simulink library "powerlib_modelsV2"  (Simulink 6.0)
settings: Solver=ode45  SolverMode=SingleTasking  StartTime=0.0  StopTime=10.0  RelTol=1e-3
values from neighbouring files (symbols this model uses):
  Ts = get(handles.edit1,'string')    [powergui.m]
undefined symbols (not defined in the file or in its folder): A, Ac, B, Bc, C, Cc, Cs, Current, damp, Dc, Dd, DiscIntNeverNeededParam, dref, dwo, exc, F, fb, gate, GH, GHd, GI, GId, GL, GLd, H, HT, hyd, ib, ib2, io, isfinite, j, K, Kd, Kg, L, Lad, Laq, lim, LIM, Ll, Llfd, Llkd, Llkq1, Llkq2, Llr, Lls, LowerFlux, N, N2, Nb, Nb2, nb_arm, p, Par_HarmoA_pu, Par_HarmoB_pu, Par_Timing_Harmo, Par_Timing_Variation, Par_Vps, Pb ... (+57)
libraries: powerlib_extras x14
(part 8 of 11)

== system powerlib_modelsV2/Discrete/MBPSS/Transfer function for detailed model (IF) ==
  On : Inport  Port=1  LatchInput=off
  "IFpos " : Inport  Port=2  LatchInput=off
  "IFneg " : Inport  Port=3  LatchInput=off
  Switch1 : Switch  Threshold=0.5  InputSameDT=on
  Switch2 : Switch  Threshold=0.5  InputSameDT=on
  Transfer functions for detailed stabilizer : Subsystem  TreatAsAtomicUnit=on
  Transfer functions for detailed stabilizer1 : Subsystem  TreatAsAtomicUnit=on
  IFpos : Outport
  IFneg : Outport  Port=2
  wires:
  Transfer functions for detailed stabilizer/1(Out1) -> Switch1/1
  "IFpos "/1 -> Transfer functions for detailed stabilizer/1(In1), Switch1/3
  Switch1/1 -> IFpos/1
  "IFneg "/1 -> Switch2/3, Transfer functions for detailed stabilizer1/1(In1)
  Switch2/1 -> IFneg/1
  Transfer functions for detailed stabilizer1/1(Out1) -> Switch2/1
  On/1 -> Transfer functions for detailed stabilizer/Enable, Switch1/2, Switch2/2, Transfer functions for detailed stabilizer1/Enable

== system powerlib_modelsV2/Discrete/MBPSS/Transfer function for detailed model (LF) ==
  On : Inport  Port=1  LatchInput=off
  "LFpos " : Inport  Port=2  LatchInput=off
  "LFneg " : Inport  Port=3  LatchInput=off
  Switch1 : Switch  Threshold=0.5  InputSameDT=on
  Switch2 : Switch  Threshold=0.5  InputSameDT=on
  Transfer functions for detailed stabilizer : Subsystem  TreatAsAtomicUnit=on
  Transfer functions for detailed stabilizer1 : Subsystem  TreatAsAtomicUnit=on
  LFpos : Outport
  LFneg : Outport  Port=2
  wires:
  On/1 -> Transfer functions for detailed stabilizer1/Enable, Switch2/2, Switch1/2, Transfer functions for detailed stabilizer/Enable
  Transfer functions for detailed stabilizer1/1(Out1) -> Switch2/1
  Switch2/1 -> LFneg/1
  "LFneg "/1 -> Transfer functions for detailed stabilizer1/1(In1), Switch2/3
  Switch1/1 -> LFpos/1
  "LFpos "/1 -> Switch1/3, Transfer functions for detailed stabilizer/1(In1)
  Transfer functions for detailed stabilizer/1(Out1) -> Switch1/1

== system powerlib_modelsV2/Discrete/PM_synchronous_machine/abc2qd ==
  note: This subsystem converts Vab and Vbc to Vd,Vq. The sine and cosine com-
      | puted here are sent to the inverse transformation subsystem dq2abc.
  Vab,Vbc : Inport  Port=1  LatchInput=off
  the : Inport  Port=2  LatchInput=off
  Elementary Math : ElementaryMath
  Elementary Math1 : ElementaryMath  Operator=cos
  Fcn2 : Fcn  Expr=(u[4]*(2*u[1]+u[2]) + (sqrt3*u[2]*u[3])) * one_third
  Fcn3 : Fcn  Expr=(u[3]*(2*u[1]+u[2]) + (-sqrt3*u[2]*u[4])) * one_third
  Mux1 : Mux  Inputs=[ 2 2 ]
  Mux2 : Mux  Inputs=2
  Mux3 : Mux  Inputs=2
  s,c : Outport  InitialOutput=0
  vq,vd : Outport  Port=2  InitialOutput=0
  wires:
  Mux1/1 -> Fcn2/1, Fcn3/1
  Mux3/1 -> s,c/1, Mux1/2
  Fcn2/1 -> Mux2/1
  Fcn3/1 -> Mux2/2
  Mux2/1 -> vq,vd/1
  Vab,Vbc/1 -> Mux1/1
  Elementary Math/1 -> Mux3/1
  Elementary Math1/1 -> Mux3/2
  the/1 -> Elementary Math/1, Elementary Math1/1

== system powerlib_modelsV2/Discrete/PM_synchronous_machine/iq,id ==
  vq,vd : Inport  Port=1  LatchInput=off
  we : Inport  Port=2  LatchInput=off
  Demux : Demux  Outputs=2
  Mux : Mux  Inputs=2
  id : Subsystem
  iq : Subsystem
  iq,id : Outport  InitialOutput=0
  wires:
  we/1 -> iq/2(we), id/2(we)
  id/1(id) -> Mux/2, iq/3(id)
  iq/1(iq) -> Mux/1, id/1(iq)
  Demux/2 -> id/3(vd)
  Demux/1 -> iq/1(vq)
  vq,vd/1 -> Demux/1
  Mux/1 -> iq,id/1

== system powerlib_modelsV2/Discrete/PM_synchronous_machine/mec ==
  Tm : Inport  Port=1  LatchInput=off
  iq,id : Inport  Port=2  LatchInput=off
  Discrete-Time Integrator : DiscreteIntegrator  SampleTime=Ts  SaturateOnIntegerOverflow=on  ICPrevOutput=DiscIntNeverNeededParam  ICPrevScaledInput=DiscIntNeverNeededParam
  Discrete-Time Integrator1 : DiscreteIntegrator  SampleTime=Ts  SaturateOnIntegerOverflow=on  ICPrevOutput=DiscIntNeverNeededParam  ICPrevScaledInput=DiscIntNeverNeededParam
  Gain : Gain  Gain=p  SaturateOnIntegerOverflow=on
  Gain1 : Gain  Gain=1/p  SaturateOnIntegerOverflow=on
  Gain2 : Gain  Gain=1/J  SaturateOnIntegerOverflow=on
  Gain3 : Gain  Gain=F  SaturateOnIntegerOverflow=on
  Mux1 : Mux  Inputs=3
  Sum : Sum  Inputs=-+-  SaturateOnIntegerOverflow=on  InputSameDT=on
  Te : Fcn  Expr=1.5*p*(lam*u(1)+(Ld-Lq)*u(1)*u(2))
  we : Outport  InitialOutput=0
  the : Outport  Port=2  InitialOutput=0
  w,th,Te : Outport  Port=3  InitialOutput=0
  wires:
  Discrete-Time Integrator1/1 -> Gain1/1, the/1
  Gain1/1 -> Mux1/2
  iq,id/1 -> Te/1
  Gain/1 -> we/1, Discrete-Time Integrator1/1
  Discrete-Time Integrator/1 -> Mux1/1, Gain3/1, Gain/1
  Gain2/1 -> Discrete-Time Integrator/1
  Sum/1 -> Gain2/1
  Tm/1 -> Sum/1
  Te/1 -> Mux1/3, Sum/2
  Mux1/1 -> w,th,Te/1
  Gain3/1 -> Sum/3

== system powerlib_modelsV2/Discrete/PM_synchronous_machine/qd2abc ==
  s,c : Inport  Port=1  LatchInput=off
  iq,id : Inport  Port=2  LatchInput=off
  Fcn : Fcn  Expr=u[3]*u[2] + u[4]*u[1]
  Fcn1 : Fcn  Expr=(u[2]*(-u[3]-sqrt3*u[4]) + u[1]*(sqrt3*u[3]-u[4]))*0.5
  Mux : Mux  Inputs=[2,2]
  Mux2 : Mux  Inputs=3
  Sum : Sum  Orientation=down  Inputs=--  SaturateOnIntegerOverflow=on  InputSameDT=on
  is : Outport  InitialOutput=0
  wires:
  Mux/1 -> Fcn/1, Fcn1/1
  s,c/1 -> Mux/1
  iq,id/1 -> Mux/2
  Sum/1 -> Mux2/3
  Fcn/1 -> Mux2/1, Sum/2
  Fcn1/1 -> Mux2/2, Sum/1
  Mux2/1 -> is/1

== system powerlib_modelsV2/Discrete/PSS/Lead-Lag #1 ==
  In1 : Inport  Port=1  LatchInput=off
  Discrete State-Space : DiscreteStateSpace  A=Ad  B=Bd  C=Cd  D=Dd  X0=x0d  SampleTime=Ts
  Out1 : Outport
  wires:
  Discrete State-Space/1 -> Out1/1
  In1/1 -> Discrete State-Space/1

== system powerlib_modelsV2/Discrete/PSS/Lead-Lag #2 ==
  In1 : Inport  Port=1  LatchInput=off
  Discrete State-Space : DiscreteStateSpace  A=Ad  B=Bd  C=Cd  D=Dd  X0=x0d  SampleTime=Ts
  Out1 : Outport
  wires:
  Discrete State-Space/1 -> Out1/1
  In1/1 -> Discrete State-Space/1

== system powerlib_modelsV2/Discrete/PSS/Sensor  ==
  In : Inport  Port=1  LatchInput=off
  Discrete State-Space : DiscreteStateSpace  A=Ad  B=Bd  C=Cd  D=Dd  X0=x0d  SampleTime=Ts
  Out : Outport  InitialOutput=0
  wires:
  Discrete State-Space/1 -> Out/1
  In/1 -> Discrete State-Space/1

== system powerlib_modelsV2/Discrete/PSS/Wash-out  ==
  In : Inport  Port=1  LatchInput=off
  Discrete State-Space : DiscreteStateSpace  A=Ad  B=Bd  C=Cd  D=Dd  X0=x0d  SampleTime=Ts
  Out : Outport  InitialOutput=0
  wires:
  Discrete State-Space/1 -> Out/1
  In/1 -> Discrete State-Space/1

== system powerlib_modelsV2/Discrete/Three-Level Bridge/2-level GTO-IGBT Bridge  Logic (modified) ==
  note: Note 3: See Sw3 logic
  note: Diode Logic :
      | 1) Diodes are blocked when complementary GTOs are switched on
  v : Inport  Port=1  LatchInput=off
  g : Inport  Port=2  LatchInput=off
  Block12 : Inport  Port=3  LatchInput=off
  Trig12 : Inport  Port=4  LatchInput=off
  Data Type  Conversion2 : DataTypeConversion  SaturateOnIntegerOverflow=on  RndMeth=Zero
  Data Type  Conversion4 : DataTypeConversion  SaturateOnIntegerOverflow=on  RndMeth=Zero
  Demux1 : Demux  Outputs=[nb_arm nb_arm]
  Diode Logic : Subsystem
  GTO Logic : Subsystem
  G_D : Logic  Operator=OR
  G_D2 : Logic  Operator=NOT
  G_D3 : Logic  Operator=OR
  G_D4 : Logic  Operator=OR
  Gain : Gain  Orientation=up  Gain=-1  SaturateOnIntegerOverflow=on
  Gain1 : Gain  Gain=2  SaturateOnIntegerOverflow=on
  Note 3 : Logic
  Select_Block3 : Selector  Elements=Block3Elements  InputPortWidth=nb_switch
  Select_Vsw : Selector  Elements=VswElements  InputPortWidth=nb_arm*3
  Unit Delay3 : UnitDelay  SampleTime=Ts
  Unit Delay9 : UnitDelay  SampleTime=Ts
  "Vf " : Subsystem
  status : Outport
  Vf : Outport  Port=2
  Block3 : Outport  Port=3
  status_GTO : Outport  Port=4
  wires:
  G_D3/1 -> Block3/1
  Gain1/1 -> Unit Delay9/1
  G_D2/1 -> Note 3/2
  Block12/1 -> G_D2/1
  Diode Logic/1(status) -> Note 3/1
  Diode Logic/2(block) -> Select_Block3/1
  Gain/1 -> Diode Logic/1(Vak)
  v/1 -> Select_Vsw/1
  "Vf "/1(Vf) -> Gain1/1
  GTO Logic/1(status) -> G_D/2, Diode Logic/2(G), "Vf "/1(status_GTO), status_GTO/1
  g/1 -> Data Type  Conversion4/1
  Data Type  Conversion4/1 -> GTO Logic/2(G)
  Unit Delay3/1 -> status/1
  G_D/1 -> Data Type  Conversion2/1
  Data Type  Conversion2/1 -> Unit Delay3/1
  Unit Delay9/1 -> Vf/1
  G_D4/1 -> G_D/1
  Note 3/1 -> G_D4/1
  Trig12/1 -> G_D4/2
  Select_Vsw/1 -> Gain/1, GTO Logic/1(Vak)
  Select_Block3/1 -> Demux1/1
  Demux1/1 -> G_D3/1
  Demux1/2 -> G_D3/2

== system powerlib_modelsV2/Discrete/Three-Level Bridge/Input ==
  note: This block is required when the "pulses" input is not connected
  In : Inport  Port=1  LatchInput=off
  Constant : Constant
  require : Logic  OutDataTypeMode=Specify via dialog  LogicDataType=float('double')
  Out : Outport
  wires:
  Constant/1 -> require/2
  In/1 -> require/1
  require/1 -> Out/1

== system powerlib_modelsV2/Discrete/Three-Level Bridge/SubSystem ==
  note: D5, D6 : Clamping diodes
  note: - Vdc ------------
  note: N ----
  note: -[Sw3]-----
  note: |
      | |
      | |
      | [Q1 - D1]
      | |
      | |
  note: |
      | |
      | [Q2 - D2]
      | |
      | |
  note: |
      | |
      | [Q3 - D3]
      | |
      | |
  note: |
      | |
      | [Q4 - D4]
      | |
      | |
      | |
  note: -------[D5]-->-------
  note: -----<-[D6]---------
  note: ------------ A
  note: |
      | |
      | |
      | |
      | |
      | |
      | |
      | |
      | |
      | |
      | |
  note: N ----------
  note: - Vdc--------------------------
  note: + Vdc --------------------------
  note: ---------- A
  note: + Vdc ------------
  note: |
      | |
      | |
      | |
      | |
      | [Sw1]
      | |
      | |
      | |
      | |
  note: |
      | |
      | |
      | |
      | |
      | [Sw2]
      | |
      | |
      | |
      | |
  note: <======>
  note: (or B or C)
  note: (or B or C)

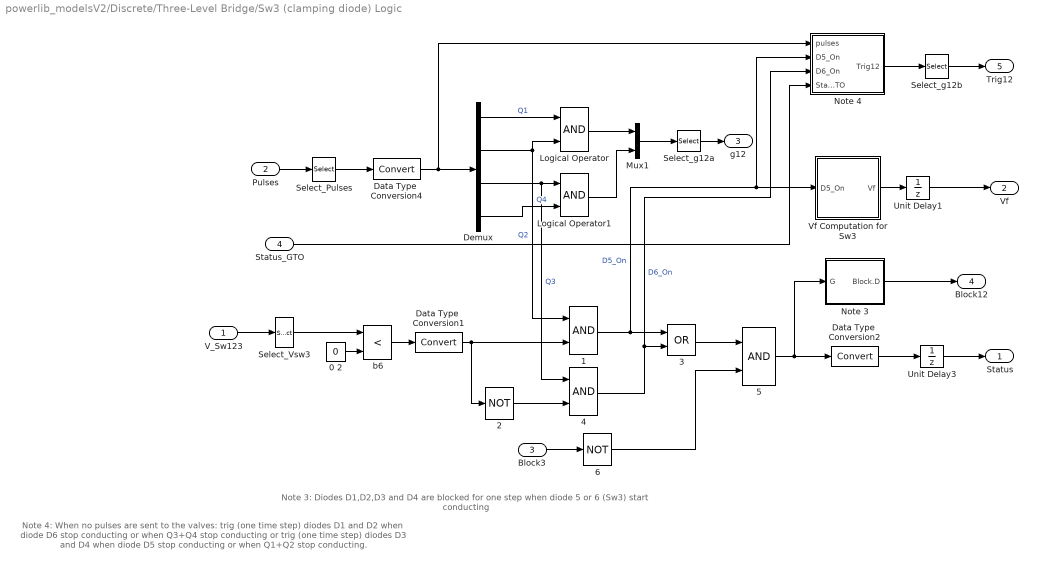
== system powerlib_modelsV2/Discrete/Three-Level Bridge/Sw3 (clamping diode) Logic ==
  note: Note 3: Diodes D1,D2,D3 and D4 are blocked for one step when diode 5 or 6 (Sw3) start conducting
  note: Note 4: When no pulses are sent to the valves:
      | trig (one time step) diodes D1 and D2 when diode D6 stop conducting or when Q3+Q4 stop conducting
      | or trig (one time step) diodes D3 and D4 when diode D5 stop conducting or when Q1+Q2 stop conducting.
  V_Sw123 : Inport  Port=1  LatchInput=off
  Pulses : Inport  Port=2  LatchInput=off
  Block3 : Inport  Port=3  LatchInput=off
  Status_GTO : Inport  Port=4  LatchInput=off
  0 2 : Constant  Value=0
  1 : Logic
  2 : Logic  Operator=NOT
  3 : Logic  Operator=OR
  4 : Logic
  5 : Logic
  6 : Logic  Operator=NOT
  Data Type  Conversion1 : DataTypeConversion  SaturateOnIntegerOverflow=on  RndMeth=Zero
  Data Type  Conversion2 : DataTypeConversion  SaturateOnIntegerOverflow=on  RndMeth=Zero
  Data Type  Conversion4 : DataTypeConversion  SaturateOnIntegerOverflow=on  RndMeth=Zero
  Demux : Demux  Outputs=[nb_arm nb_arm nb_arm nb_arm]
  Logical Operator : Logic
  Logical Operator1 : Logic
  Mux1 : Mux  Inputs=[nb_arm nb_arm]
  Note 3 : Subsystem
  Note 4 : Subsystem
  Select_Pulses : Selector  Elements=PulseElements  InputPortWidth=nb_arm*4
  Select_Vsw3 : Selector  Elements=Vsw3Elements  InputPortWidth=nb_arm*3
  Select_g12a : Selector  Elements=g12Elements  InputPortWidth=nb_arm*2
  Select_g12b : Selector  Elements=g12Elements  InputPortWidth=nb_arm*2
  Unit Delay1 : UnitDelay  SampleTime=Ts
  Unit Delay3 : UnitDelay  SampleTime=Ts
  Vf Computation for Sw3 : Subsystem
  b6 : RelationalOperator  Operator=<  InputSameDT=on
  Status : Outport
  Vf : Outport  Port=2
  g12 : Outport  Port=3
  Block12 : Outport  Port=4
  Trig12 : Outport  Port=5
  wires:
  Select_g12b/1 -> Trig12/1
  Select_g12a/1 -> g12/1
  Logical Operator/1 -> Mux1/1
  Select_Vsw3/1 -> b6/1
  5/1 -> Note 3/1(G), Data Type  Conversion2/1
  Note 3/1(Block.D) -> Block12/1
  Block3/1 -> 6/1
  Unit Delay3/1 -> Status/1
  2/1 -> 4/2
  V_Sw123/1 -> Select_Vsw3/1
  0 2/1 -> b6/2
  Pulses/1 -> Select_Pulses/1
  Mux1/1 -> Select_g12a/1
  Vf Computation for Sw3/1(Vf) -> Unit Delay1/1
  Unit Delay1/1 -> Vf/1
  Data Type  Conversion4/1 -> Demux/1, Note 4/1(pulses)
  Demux/1 -> Logical Operator/1  "Q1"
  Demux/2 -> Logical Operator/2, 1/1  "Q2"
  Demux/3 -> 4/1, Logical Operator1/1  "Q3"
  Demux/4 -> Logical Operator1/2  "Q4"
  Logical Operator1/1 -> Mux1/2
  b6/1 -> Data Type  Conversion1/1
  Data Type  Conversion1/1 -> 1/2, 2/1
  4/1 -> 3/2, Note 4/3(D6_On)  "D6_On"
  1/1 -> 3/1, Vf Computation for Sw3/1(D5_On), Note 4/2(D5_On)  "D5_On"
  3/1 -> 5/1
  6/1 -> 5/2
  Data Type  Conversion2/1 -> Unit Delay3/1
  Note 4/1(Trig12) -> Select_g12b/1
  Select_Pulses/1 -> Data Type  Conversion4/1
  Status_GTO/1 -> Note 4/4(Status_GTO)

== system powerlib_modelsV2/Discrete/asynchronous_machine/Mechanical ==
  Tm : Inport  Port=1  LatchInput=off
  phis,is : Inport  Port=2  LatchInput=off
  1\p : Gain  Gain=1/p  SaturateOnIntegerOverflow=on
  1_2H : Gain  Gain=1/(2*H)  SaturateOnIntegerOverflow=on
  1_Tb2 : Gain  Gain=1/Tb2  SaturateOnIntegerOverflow=on
  Discrete-Time Integrator : DiscreteIntegrator  InitialCondition=wmo  SampleTime=Ts  SaturateOnIntegerOverflow=on  ICPrevOutput=DiscIntNeverNeededParam  ICPrevScaledInput=DiscIntNeverNeededParam
  Discrete-Time Integrator1 : DiscreteIntegrator  InitialCondition=tho  SampleTime=Ts  SaturateOnIntegerOverflow=on  ICPrevOutput=DiscIntNeverNeededParam  ICPrevScaledInput=DiscIntNeverNeededParam
  F : Gain  Orientation=left  Gain=F  SaturateOnIntegerOverflow=on
  Mux3 : Mux  Inputs=2
  Mux4 : Mux  Inputs=3
  Product1 : Product  Inputs=1  SaturateOnIntegerOverflow=on  InputSameDT=on
  Product2 : Product  Inputs=1  SaturateOnIntegerOverflow=on  InputSameDT=on
  Selector : Selector  Elements=[1 4]  InputPortWidth=4
  Selector1 : Selector  Elements=[2 3]  InputPortWidth=4
  Sum : Sum  Inputs=-+-  SaturateOnIntegerOverflow=on  InputSameDT=on
  Sum1 : Sum  Inputs=|-+  SaturateOnIntegerOverflow=on  InputSameDT=on
  web_psb : Gain  Gain=web_psb  SaturateOnIntegerOverflow=on
  w,Te,thr : Outport
  thr,wr : Outport  Port=2
  wires:
  Discrete-Time Integrator1/1 -> Mux3/1, 1\p/1
  1\p/1 -> Mux4/3
  web_psb/1 -> Discrete-Time Integrator1/1
  Sum1/1 -> Sum/2, Mux4/2
  1_Tb2/1 -> Sum/1
  F/1 -> Sum/3
  Discrete-Time Integrator/1 -> web_psb/1, Mux4/1, Mux3/2, F/1
  1_2H/1 -> Discrete-Time Integrator/1
  Sum/1 -> 1_2H/1
  Tm/1 -> 1_Tb2/1
  Mux3/1 -> thr,wr/1
  Mux4/1 -> w,Te,thr/1
  Product1/1 -> Sum1/1
  Product2/1 -> Sum1/2
  phis,is/1 -> Selector/1, Selector1/1
  Selector1/1 -> Product2/1
  Selector/1 -> Product1/1

== system powerlib_modelsV2/Discrete/asynchronous_machine/Mutual fluxes ==
  phiqr,phidr : Inport  Port=1  LatchInput=off
  phiqs,phids : Inport  Port=2  LatchInput=off
  1\Llr : Gain  Gain=1/Llr  SaturateOnIntegerOverflow=on
  1\Llr1 : Gain  Gain=Laq  SaturateOnIntegerOverflow=on
  1\Llr2 : Gain  Gain=Lad  SaturateOnIntegerOverflow=on
  1\Lls : Gain  Gain=1/Lls  SaturateOnIntegerOverflow=on
  Demux1 : Demux  Outputs=2
  Demux2 : Demux  Outputs=2
  Mux3 : Mux  Inputs=2
  Sum : Sum  Inputs=|++  SaturateOnIntegerOverflow=on  InputSameDT=on
  Sum1 : Sum  Inputs=++|  SaturateOnIntegerOverflow=on  InputSameDT=on
  phimq,phimd : Outport
  wires:
  Mux3/1 -> phimq,phimd/1
  1\Llr2/1 -> Mux3/2
  1\Llr1/1 -> Mux3/1
  Demux1/2 -> Sum1/1
  Demux2/2 -> Sum1/2
  Demux2/1 -> Sum/2
  1\Lls/1 -> Demux2/1
  Sum/1 -> 1\Llr1/1
  Demux1/1 -> Sum/1
  1\Llr/1 -> Demux1/1
  phiqr,phidr/1 -> 1\Llr/1
  phiqs,phids/1 -> 1\Lls/1
  Sum1/1 -> 1\Llr2/1

== system powerlib_modelsV2/Discrete/asynchronous_machine/Rotor ==
  vqr,vdr : Inport  Port=1  LatchInput=off
  w-wr : Inport  Port=2  LatchInput=off
  phimq,phimd : Inport  Port=3  LatchInput=off
  1\Llr : Gain  Gain=1/Llr  SaturateOnIntegerOverflow=on
  1\Llr1 : Gain  Gain=Rr  SaturateOnIntegerOverflow=on
  1\Llr2 : Gain  Gain=1/Llr  SaturateOnIntegerOverflow=on
  1\Llr3 : Gain  Gain=Rr  SaturateOnIntegerOverflow=on
  Demux : Demux  Outputs=2
  Demux1 : Demux  Outputs=2
  Discrete-Time Integrator : DiscreteIntegrator  InitialCondition=phirqo  SampleTime=Ts  SaturateOnIntegerOverflow=on  ICPrevOutput=DiscIntNeverNeededParam  ICPrevScaledInput=DiscIntNeverNeededParam
  Discrete-Time Integrator1 : DiscreteIntegrator  InitialCondition=phirdo  SampleTime=Ts  SaturateOnIntegerOverflow=on  ICPrevOutput=DiscIntNeverNeededParam  ICPrevScaledInput=DiscIntNeverNeededParam
  Mux2 : Mux  Inputs=2
  Mux3 : Mux  Inputs=2
  Product : Product  SaturateOnIntegerOverflow=on  InputSameDT=on
  Product1 : Product  Orientation=left  SaturateOnIntegerOverflow=on  InputSameDT=on
  Sum1 : Sum  Inputs=++-||  SaturateOnIntegerOverflow=on  InputSameDT=on
  Sum2 : Sum  Inputs=+--  SaturateOnIntegerOverflow=on  InputSameDT=on
  Sum3 : Sum  Inputs=+-|  SaturateOnIntegerOverflow=on  InputSameDT=on
  Sum4 : Sum  Inputs=-+|  SaturateOnIntegerOverflow=on  InputSameDT=on
  web1 : Gain  Gain=web_psb  SaturateOnIntegerOverflow=on
  web_psb : Gain  Gain=web_psb  SaturateOnIntegerOverflow=on
  iqr,idr : Outport
  phiqr,phidr : Outport  Port=2
  wires:
  Mux3/1 -> phiqr,phidr/1
  Discrete-Time Integrator/1 -> Mux3/1, Product1/2, Sum3/1  "phiqr"
  web1/1 -> Discrete-Time Integrator1/1
  Sum1/1 -> web1/1
  w-wr/1 -> Product/2, Product1/1
  Product/1 -> Sum2/2
  web_psb/1 -> Discrete-Time Integrator/1
  Sum2/1 -> web_psb/1
  Discrete-Time Integrator1/1 -> Sum4/2, Product/1, Mux3/2
  vqr,vdr/1 -> Demux/1
  Product1/1 -> Sum1/1
  Demux/2 -> Sum1/2
  1\Llr3/1 -> Sum1/3
  1\Llr2/1 -> 1\Llr3/1, Mux2/2  "idr"
  Sum4/1 -> 1\Llr2/1
  Demux1/2 -> Sum4/1
  Mux2/1 -> iqr,idr/1
  1\Llr/1 -> Mux2/1, 1\Llr1/1  "iqr"
  1\Llr1/1 -> Sum2/3
  Sum3/1 -> 1\Llr/1
  Demux/1 -> Sum2/1
  Demux1/1 -> Sum3/2
  phimq,phimd/1 -> Demux1/1

== system powerlib_modelsV2/Discrete/asynchronous_machine/Stator ==
  phimq,phimd : Inport  Port=1  LatchInput=off
  vqs,vds : Inport  Port=2  LatchInput=off
  w : Inport  Port=3  LatchInput=off
  1\Llr : Gain  Gain=1/Lls  SaturateOnIntegerOverflow=on
  1\Llr1 : Gain  Gain=Rs  SaturateOnIntegerOverflow=on
  1\Llr2 : Gain  Gain=1/Lls  SaturateOnIntegerOverflow=on
  1\Llr3 : Gain  Gain=Rs  SaturateOnIntegerOverflow=on
  Demux : Demux  Outputs=2
  Demux1 : Demux  Outputs=2
  Discrete-Time Integrator : DiscreteIntegrator  InitialCondition=phisqo  SampleTime=Ts  SaturateOnIntegerOverflow=on  ICPrevOutput=DiscIntNeverNeededParam  ICPrevScaledInput=DiscIntNeverNeededParam
  Discrete-Time Integrator1 : DiscreteIntegrator  InitialCondition=phisdo  SampleTime=Ts  SaturateOnIntegerOverflow=on  ICPrevOutput=DiscIntNeverNeededParam  ICPrevScaledInput=DiscIntNeverNeededParam
  Mux2 : Mux  Inputs=2
  Mux3 : Mux  Inputs=2
  Mux4 : Mux  Inputs=2
  Product : Product  SaturateOnIntegerOverflow=on  InputSameDT=on
  Product1 : Product  SaturateOnIntegerOverflow=on  InputSameDT=on
  Sum1 : Sum  Inputs=++-||  SaturateOnIntegerOverflow=on  InputSameDT=on
  Sum2 : Sum  Inputs=--+  SaturateOnIntegerOverflow=on  InputSameDT=on
  Sum3 : Sum  Inputs=-+  SaturateOnIntegerOverflow=on  InputSameDT=on
  Sum4 : Sum  Inputs=+-|  SaturateOnIntegerOverflow=on  InputSameDT=on
  web1 : Gain  Gain=web_psb  SaturateOnIntegerOverflow=on
  web_psb : Gain  Gain=web_psb  SaturateOnIntegerOverflow=on
  phiqs,phids : Outport
  iqs,ids : Outport  Port=2
  phis,is : Outport  Port=3
  wires:
  phimq,phimd/1 -> Demux1/1
  Demux1/1 -> Sum4/2
  Sum4/1 -> 1\Llr/1
  1\Llr/1 -> Mux2/1, 1\Llr1/1  "iqs"
  1\Llr1/1 -> Sum2/1
  vqs,vds/1 -> Demux/1
  Sum2/1 -> web_psb/1
  Demux/1 -> Sum2/3
  Product/1 -> Sum2/2
  web_psb/1 -> Discrete-Time Integrator/1
  Discrete-Time Integrator/1 -> Mux3/1, Product1/2, Sum4/1
  Mux2/1 -> iqs,ids/1, Mux4/2
  w/1 -> Product/1, Product1/1
  Demux1/2 -> Sum3/1
  Sum3/1 -> 1\Llr2/1
  1\Llr2/1 -> 1\Llr3/1, Mux2/2  "ids"
  1\Llr3/1 -> Sum1/3
  web1/1 -> Discrete-Time Integrator1/1
  Sum1/1 -> web1/1
  Discrete-Time Integrator1/1 -> Product/2, Sum3/2, Mux3/2
  Demux/2 -> Sum1/2
  Product1/1 -> Sum1/1
  Mux3/1 -> phiqs,phids/1, Mux4/1
  Mux4/1 -> phis,is/1

== system powerlib_modelsV2/Discrete/asynchronous_machine/abc2qd ==
  v : Inport  Port=1  LatchInput=off
  sin,cos : Inport  Port=2  LatchInput=off
  1_Vb : Gain  Gain=1/Vb  SaturateOnIntegerOverflow=on
  Constant : Constant  Orientation=down  Value=ctrl==1
  Constant1 : Constant  Orientation=down  Value=ctrl==2
  Constant2 : Constant  Orientation=down  Value=ctrl==3
  Constant3 : Constant  Orientation=down  Value=ctrl
  Constant4 : Constant  Orientation=left  Value=ctrl
  Multiport Switch : MultiPortSwitch  Inputs=3  InputSameDT=on
  Multiport Switch1 : MultiPortSwitch  Inputs=3  InputSameDT=on
  Mux : Mux  Inputs=2
  Rotor reference frame : Subsystem  TreatAsAtomicUnit=on
      mask Display: disp('Rotor\nreference\nframe')
  Stationary reference frame : Subsystem  TreatAsAtomicUnit=on
      mask Display: disp('Stationary\nreference\nframe')
  Synchronous reference frame : Subsystem  TreatAsAtomicUnit=on
      mask Display: disp('Synchronous\nreference\nframe')
  transit : Subsystem
  vqr,vdr : Outport
  vqs,vds : Outport  Port=2
  wires:
  transit/1(vr,vs) -> 1_Vb/1
  Constant4/1 -> Multiport Switch1/1
  Constant3/1 -> Multiport Switch/1
  1_Vb/1 -> Mux/1
  Mux/1 -> Synchronous reference frame/1(In1), Stationary reference frame/1(In1), Rotor reference frame/1(In1)
  sin,cos/1 -> Mux/2
  Multiport Switch/1 -> vqr,vdr/1
  Synchronous reference frame/2(vqs,vds) -> Multiport Switch1/4
  Stationary reference frame/2(vqs,vds) -> Multiport Switch1/3
  Rotor reference frame/2(vqs,vds) -> Multiport Switch1/2
  Synchronous reference frame/1(vqr,vdr) -> Multiport Switch/4
  Stationary reference frame/1(vqr,vdr) -> Multiport Switch/3
  Rotor reference frame/1(vqr,vdr) -> Multiport Switch/2
  Multiport Switch1/1 -> vqs,vds/1
  Constant2/1 -> Synchronous reference frame/Enable
  Constant1/1 -> Stationary reference frame/Enable
  Constant/1 -> Rotor reference frame/Enable
  v/1 -> transit/1(vu)

== system powerlib_modelsV2/Discrete/asynchronous_machine/dq2abc ==
  sin,cos : Inport  Port=1  LatchInput=off
  iqr,idr : Inport  Port=2  LatchInput=off
  iqs,ids : Inport  Port=3  LatchInput=off
  Constant : Constant  Orientation=down  Value=ctrl==1
  Constant1 : Constant  Orientation=down  Value=ctrl==2
  Constant2 : Constant  Orientation=down  Value=ctrl==3
  Constant3 : Constant  Orientation=down  Value=ctrl
  Constant4 : Constant  Orientation=left  Value=ctrl
  Multiport Switch : MultiPortSwitch  Inputs=3  InputSameDT=on
  Multiport Switch1 : MultiPortSwitch  Inputs=3  InputSameDT=on
  Mux : Mux  Inputs=3
  Mux1 : Mux  Inputs=2
  Mux2 : Mux  Inputs=2
  Mux3 : Mux  Inputs=2
  Rotor reference frame : Subsystem  TreatAsAtomicUnit=on
      mask Display: disp('Rotor\nreference\nframe')
  Selector : Selector  Elements=elements2  InputPortWidth=4
  Stationary reference frame : Subsystem  TreatAsAtomicUnit=on
      mask Display: disp('Stationary\nreference\nframe')
  Sum2 : Sum  Inputs=-  SaturateOnIntegerOverflow=on  InputSameDT=on
  Sum3 : Sum  Inputs=-  SaturateOnIntegerOverflow=on  InputSameDT=on
  Synchronous reference frame : Subsystem  TreatAsAtomicUnit=on
      mask Display: disp('Synchronous\nreference\nframe')
  ib : Gain  Gain=ib  SaturateOnIntegerOverflow=on
  irab,isab : Outport
  irabc : Outport  Port=2
  isabc : Outport  Port=3
  wires:
  Selector/1 -> irab,isab/1
  ib/1 -> Selector/1
  Mux3/1 -> isabc/1
  Sum3/1 -> Mux3/2
  Constant4/1 -> Multiport Switch1/1
  Constant3/1 -> Multiport Switch/1
  Mux1/1 -> ib/1
  Rotor reference frame/2(isa,isb) -> Multiport Switch1/2
  sin,cos/1 -> Mux/3
  Sum2/1 -> Mux2/2
  Multiport Switch1/1 -> Mux3/1, Sum3/1, Mux1/2
  Mux2/1 -> irabc/1
  Multiport Switch/1 -> Sum2/1, Mux1/1, Mux2/1
  iqr,idr/1 -> Mux/1
  iqs,ids/1 -> Mux/2
  Mux/1 -> Synchronous reference frame/1(In1), Stationary reference frame/1(In1), Rotor reference frame/1(In1)
  Synchronous reference frame/2(isa,isb) -> Multiport Switch1/4
  Stationary reference frame/2(isa,isb) -> Multiport Switch1/3
  Synchronous reference frame/1(ira,irb) -> Multiport Switch/4
  Stationary reference frame/1(ira,irb) -> Multiport Switch/3
  Rotor reference frame/1(ira,irb) -> Multiport Switch/2
  Constant2/1 -> Synchronous reference frame/Enable
  Constant1/1 -> Stationary reference frame/Enable
  Constant/1 -> Rotor reference frame/Enable

== system powerlib_modelsV2/Discrete/asynchronous_machine/sin,cos ==
  thr,wr : Inport  Port=1  LatchInput=off
  Constant : Constant  Orientation=down  Value=ctrl<3
  Constant1 : Constant  Value=ctrl
  Constant2 : Constant  Value=0
  Constant3 : Constant  Orientation=down  Value=ctrl==3
  Constant4 : Constant  Value=ctrl
  Constant5 : Constant  Value=0
  Constant6 : Constant
  Gain : Gain  Gain=-1  SaturateOnIntegerOverflow=on
  Multiport Switch : MultiPortSwitch  Inputs=3  InputSameDT=on
  Multiport Switch1 : MultiPortSwitch  Inputs=3  InputSameDT=on
  Selector : Selector  InputPortWidth=2
  Selector1 : Selector  Elements=2  InputPortWidth=2
  Switch : Switch  Threshold=0.5  InputSameDT=on
  sin(beta),cos(beta),sin(th),cos(th) : Subsystem  TreatAsAtomicUnit=on
  sin(thr),cos(thr) : Subsystem  TreatAsAtomicUnit=on
  sin,cos : Outport
  w-wr : Outport  Port=2
  w : Outport  Port=3
  wires:
  Constant/1 -> sin(thr),cos(thr)/Enable, Switch/2
  thr,wr/1 -> Selector/1, sin(beta),cos(beta),sin(th),cos(th)/1(thr,wr), Selector1/1
  Selector/1 -> sin(thr),cos(thr)/1(thr)
  Switch/1 -> sin,cos/1
  Constant3/1 -> sin(beta),cos(beta),sin(th),cos(th)/Enable
  sin(beta),cos(beta),sin(th),cos(th)/2(we-wr) -> Multiport Switch/4
  Constant1/1 -> Multiport Switch/1
  Constant2/1 -> Multiport Switch/2
  Multiport Switch/1 -> w-wr/1
  sin(thr),cos(thr)/1(sin(thr),cos(thr)) -> Switch/1
  sin(beta),cos(beta),sin(th),cos(th)/1("sin(beta),cos(beta), sin(th),cos(th)") -> Switch/3
  Gain/1 -> Multiport Switch/3  "-wr"
  Selector1/1 -> Gain/1, Multiport Switch1/2
  Constant4/1 -> Multiport Switch1/1
  Constant5/1 -> Multiport Switch1/3
  Constant6/1 -> Multiport Switch1/4
  Multiport Switch1/1 -> w/1

== system powerlib_modelsV2/Discrete/hysteresis_transformer/Hysteresis ( always in SI ) ==
  In1 : Inport  Port=1  LatchInput=off
  Hysteresis main loop + Saturation (Lower Part) : Lookup  DialogController=Simulink.DDGSource  InputValues=LowerFlux  OutputValues=Current  SaturateOnIntegerOverflow=on
  Hysteresis main loop + Saturation. (Upper Part) : Lookup  DialogController=Simulink.DDGSource  InputValues=UpperFlux  OutputValues=Current  SaturateOnIntegerOverflow=on
  Memory : Memory
  Memory1 : Memory  Orientation=down
  SI conversion2 : Gain  Gain=ib  SaturateOnIntegerOverflow=on
  Selector : Selector  Elements=2  InputPortWidth=2
  Selector1 : Selector  InputPortWidth=2
  Sign : Signum
  Sum : Sum  Inputs=|+-  SaturateOnIntegerOverflow=on  InputSameDT=on
  Switch1 : Switch  InputSameDT=on
  Switch2 : Switch  Threshold=1.5  InputSameDT=on
  Tr : Display
  pu conversion : Gain  Gain=fb  SaturateOnIntegerOverflow=on
  sfun_psbtransfosat : S-Function  FunctionName=sfun_test  Parameters=fluxinit*fb,HT,indice,Ts,Tolerances,initialslope
  Out1 : Outport
  wires:
  Memory1/1 -> pu conversion/1
  Hysteresis main loop + Saturation (Lower Part)/1 -> Switch1/1  "courbe principale + Saturation, partie du bas, le flux est en monte, donc sens positif"
  In1/1 -> Hysteresis main loop + Saturation (Lower Part)/1, Memory/1, Sum/1, Memory1/1, Hysteresis main loop + Saturation. (Upper Part)/1
  Hysteresis main loop + Saturation. (Upper Part)/1 -> Switch1/3  "courbe principale + Saturation, partie superieure, le flux est en descente, donc sens negatif"
  Memory/1 -> Sum/2  "precedent"
  Sign/1 -> Switch1/2  "sens du flux"
  pu conversion/1 -> sfun_psbtransfosat/1
  sfun_psbtransfosat/1 -> Selector/1, Selector1/1
  Switch2/1 -> Out1/1
  Switch1/1 -> Switch2/3
  Selector/1 -> Switch2/2, Tr/1  "Tr"
  Selector1/1 -> SI conversion2/1
  SI conversion2/1 -> Switch2/1  "Boucles internes"
  Sum/1 -> Sign/1

== system powerlib_modelsV2/Discrete/simplified_sync_mach/Subsystem ==
  i : Inport  Port=1  LatchInput=off
  v : Inport  Port=2  LatchInput=off
  e : Inport  Port=3  LatchInput=off
  theta : Inport  Port=4  LatchInput=off
  wm : Inport  Port=5  LatchInput=off
  Pe : Inport  Port=6  LatchInput=off
  Gain : Gain  Gain=[ ib2*ones(3,1); Vb3*ones(6,1); 1; Nb; Pb ]  SaturateOnIntegerOverflow=on
  Mux : Mux  Inputs=[ 3 3 3 1 1 1 ]
  * : Outport  InitialOutput=0
  wires:
  i/1 -> Mux/1
  v/1 -> Mux/2
  e/1 -> Mux/3
  theta/1 -> Mux/4
  wm/1 -> Mux/5
  Pe/1 -> Mux/6
  Mux/1 -> Gain/1
  Gain/1 -> */1

== system powerlib_modelsV2/Discrete/simplified_sync_mach/Vt ==
  note: This subsystem either converts 2 line-to-line voltages to 3 line-to-neutral voltages (internal neutral)
      | and computes floating neutral voltage or directly passes Van,Vbn,Vcn if 4-wire connection.
  V : Inport  Port=1  LatchInput=off
  1_Vb : Gain  Gain=1/Vb  SaturateOnIntegerOverflow=on
  Constant : Constant  Orientation=down  Value=v6==1
  Constant1 : Constant  Value=0
  Constant2 : Constant  Value=0
  Data Type  Conversion : DataTypeConversion  Orientation=left  SaturateOnIntegerOverflow=on  RndMeth=Zero
  Data Type  Conversion1 : DataTypeConversion  SaturateOnIntegerOverflow=on  RndMeth=Zero
  Fcn : Fcn  Expr=u[1]
  Fcn1 : Fcn  Expr=u[2]
  Fcn2 : Fcn  Expr=u[3]
  Gain : Gain  Gain=1/3  SaturateOnIntegerOverflow=on
  LL2LN : Subsystem  TreatAsAtomicUnit=on
  Logical Operator : Logic  Operator=NOT
  Mux : Mux  Inputs=2
  Mux1 : Mux  Inputs=3
  Product : Product  SaturateOnIntegerOverflow=on  InputSameDT=on
  Sum : Sum  Inputs=+  SaturateOnIntegerOverflow=on  InputSameDT=on
  Sum1 : Sum  Inputs=|++  SaturateOnIntegerOverflow=on  InputSameDT=on
  Switch2 : Switch  Threshold=0.5  InputSameDT=on
  Vn : Outport  InitialOutput=0
  Vabc : Outport  Port=2  InitialOutput=0
  wires:
  Data Type  Conversion1/1 -> Product/1
  Logical Operator/1 -> Data Type  Conversion1/1
  Data Type  Conversion/1 -> Logical Operator/1
  1_Vb/1 -> Mux/1, LL2LN/1(In1)
  V/1 -> 1_Vb/1
  Product/1 -> Sum1/2
  Mux1/1 -> Product/2
  Fcn2/1 -> Mux1/3
  Fcn1/1 -> Mux1/2
  Fcn/1 -> Mux1/1
  Mux/1 -> Fcn2/1, Fcn1/1, Fcn/1
  Constant1/1 -> Mux/2
  Sum1/1 -> Vabc/1
  LL2LN/1(Out1) -> Sum1/1, Sum/1
  Constant/1 -> Data Type  Conversion/1, LL2LN/Enable, Switch2/2
  Switch2/1 -> Vn/1
  Constant2/1 -> Switch2/3
  Gain/1 -> Switch2/1
  Sum/1 -> Gain/1

== system powerlib_modelsV2/Discrete/simplified_sync_mach/Z ==
  note: This subsystem models the internal impedance of
      | the machine, which consists of  a series RL circuit.
  e : Inport  Port=1  LatchInput=off
  v : Inport  Port=2  LatchInput=off
  1/L : Gain  Gain=web_psb/L  SaturateOnIntegerOverflow=on
  Discrete-Time Integrator : DiscreteIntegrator  IntegratorMethod=Integration: Trapezoidal  InitialCondition=io  SampleTime=Ts  SaturateOnIntegerOverflow=on  ICPrevOutput=DiscIntNeverNeededParam  ICPrevScaledInput=DiscIntNeverNeededParam
  R : Gain  Orientation=left  Gain=R  SaturateOnIntegerOverflow=on
  Sum5 : Sum  Inputs=-+-  SaturateOnIntegerOverflow=on  InputSameDT=on
  Unit Delay : UnitDelay  X0=io  SampleTime=Ts
  i : Outport  InitialOutput=0
  wires:
  e/1 -> Sum5/2
  R/1 -> Sum5/1
  Sum5/1 -> 1/L/1
  v/1 -> Sum5/3
  1/L/1 -> Discrete-Time Integrator/1
  Discrete-Time Integrator/1 -> Unit Delay/1
  Unit Delay/1 -> R/1, i/1

== system powerlib_modelsV2/Discrete/simplified_sync_mach/gen ==
  note: This subsystem generates the 3 line-to-neutral voltages inside the machine.
  theta : Inport  Port=1  LatchInput=off
  E : Inport  Port=2  LatchInput=off
  Vn : Inport  Port=3  LatchInput=off
  1_Vb2 : Gain  Gain=1/Vb2  SaturateOnIntegerOverflow=on
  Mux : Mux  Inputs=3
  Product : Product  SaturateOnIntegerOverflow=on  InputSameDT=on
  Sum : Sum  Inputs=|++  SaturateOnIntegerOverflow=on  InputSameDT=on
  Sum1 : Sum  Orientation=down  Inputs=--  SaturateOnIntegerOverflow=on  InputSameDT=on
  rem(wt,2pi) : Fcn  Expr=rem(u[1],2*pi)
  sin(a) : Fcn  Expr=sin(u)
  sin(b) : Fcn  Expr=sin(u-pi23)
  e : Outport  InitialOutput=0
  wires:
  Sum/1 -> e/1
  Product/1 -> Sum/1
  Mux/1 -> Product/1
  Vn/1 -> Sum/2
  1_Vb2/1 -> Product/2
  E/1 -> 1_Vb2/1
  sin(b)/1 -> Mux/2, Sum1/1
  Sum1/1 -> Mux/3
  sin(a)/1 -> Mux/1, Sum1/2
  theta/1 -> rem(wt,2pi)/1
  rem(wt,2pi)/1 -> sin(b)/1, sin(a)/1

== system powerlib_modelsV2/Discrete/simplified_sync_mach/mechanics ==
  Pm : Inport  Port=1  LatchInput=off
  Pe : Inport  Port=2  LatchInput=off
  1_(2*H) : Gain  Gain=1/(2*H)  SaturateOnIntegerOverflow=on
  1_Pb : Gain  Gain=1/Pb  SaturateOnIntegerOverflow=on
  Discrete-Time Integrator : DiscreteIntegrator  IntegratorMethod=Integration: Trapezoidal  InitialCondition=dwo  SampleTime=Ts  SaturateOnIntegerOverflow=on  ICPrevOutput=DiscIntNeverNeededParam  ICPrevScaledInput=DiscIntNeverNeededParam
  Discrete-Time Integrator1 : DiscreteIntegrator  IntegratorMethod=Integration: Trapezoidal  InitialCondition=tho  SampleTime=Ts  SaturateOnIntegerOverflow=on  ICPrevOutput=DiscIntNeverNeededParam  ICPrevScaledInput=DiscIntNeverNeededParam
  Gain : Gain  Orientation=left  Gain=Kd  SaturateOnIntegerOverflow=on
  Mux1 : Mux  Inputs=2
  Predict : Subsystem
  Sum : Sum  SaturateOnIntegerOverflow=on  InputSameDT=on
  Sum1 : Sum  Inputs=+-  SaturateOnIntegerOverflow=on  InputSameDT=on
  Sum2 : Sum  Inputs=-+  SaturateOnIntegerOverflow=on  InputSameDT=on
  Unit Delay2 : UnitDelay  X0=dwo  SampleTime=Ts
  div : Fcn  Expr=u[2]/u[1]
      mask Display: disp('division')
  nom. speed : Constant
  web_psb : Gain  Gain=web_psb  SaturateOnIntegerOverflow=on
  theta_e : Outport  InitialOutput=0
  wm : Outport  Port=2  InitialOutput=0
  wires:
  nom. speed/1 -> Sum/1
  Discrete-Time Integrator/1 -> Unit Delay2/1
  Sum1/1 -> 1_(2*H)/1
  Gain/1 -> Sum1/2
  div/1 -> Sum1/1
  1_(2*H)/1 -> Discrete-Time Integrator/1
  Sum/1 -> web_psb/1, wm/1, Mux1/1
  Sum2/1 -> Mux1/2
  Pe/1 -> Sum2/1
  Mux1/1 -> div/1
  Discrete-Time Integrator1/1 -> theta_e/1
  web_psb/1 -> Discrete-Time Integrator1/1
  1_Pb/1 -> Sum2/2
  Pm/1 -> 1_Pb/1
  Unit Delay2/1 -> Predict/1(I)
  Predict/1(O) -> Gain/1, Sum/2

== system powerlib_modelsV2/Discrete/simplified_sync_mach/wattmeter ==
  note: This subsystem computes the total electrical
      | power delivered or absorbed by the machine.
  i : Inport  Port=1  LatchInput=off
  v : Inport  Port=2  LatchInput=off
  2_3 : Gain  Gain=2/3  SaturateOnIntegerOverflow=on
  Product : Product  SaturateOnIntegerOverflow=on  InputSameDT=on
  Sum : Sum  Inputs=+  SaturateOnIntegerOverflow=on  InputSameDT=on
  Pe : Outport  InitialOutput=0
  wires:
  2_3/1 -> Pe/1
  Sum/1 -> 2_3/1
  v/1 -> Product/2
  i/1 -> Product/1
  Product/1 -> Sum/1

== system powerlib_modelsV2/Discrete/synchronous_machine/Delta angle ==
  Vq : Inport  Port=1  PortDimensions=1  LatchInput=off
  Vd : Inport  Port=2  PortDimensions=1  LatchInput=off
  Cartesian to Polar : Subsystem
      mask Type: Cart2Polar
      mask Description:
      | Transformation from cartesian to polar coordinates.
      | [x, y] -> [r, theta]
      | 
      | r = sqrt(x^2 + y^2);
      | theta = atan(y/x);
      mask Help: Unmask this block for more help.
      mask Display: plot(0,0,100,100,[24,20,15,20,20],[85,95,85,95,20],[80,20,95,85,95,85],[70,20,20,15,20,24],[56,56,55,52,50,46],[20,26,31,35,38,42])
  Radians to Degrees : Subsystem
      mask Type: RadiansToDegrees
      mask Description:
      | Conversion from Radians to Degrees.
      | 
      | D=180/pi*R
      mask Help: This block converts from Radians to Degrees.
      mask Display: disp('R2D')
  Terminator2 : Terminator
  delta : Outport
  wires:
  Vd/1 -> Cartesian to Polar/2(y)
  Radians to Degrees/1(Degrees out) -> delta/1  "delta"
  Vq/1 -> Cartesian to Polar/1(x)
  Cartesian to Polar/1(r) -> Terminator2/1
  Cartesian to Polar/2(theta) -> Radians to Degrees/1(Radians in)

== system powerlib_modelsV2/Discrete/synchronous_machine/PQ ==
  note: P = Vd*Id + Vq*Iq
  note: Q = Vq*Id-Vd*Iq
  note: PQ Measurement:
  Vq : Inport  Port=1  PortDimensions=1  LatchInput=off
  Vd : Inport  Port=2  PortDimensions=1  LatchInput=off
  Iq : Inport  Port=3  PortDimensions=2  LatchInput=off
  Demux1 : Demux  Outputs=[1,1]
  Gain : Gain  Gain=Gain1  SaturateOnIntegerOverflow=on
  Gain1 : Gain  Gain=Gain1  SaturateOnIntegerOverflow=on
  Product{2..5} (4 alike) : Product  SaturateOnIntegerOverflow=on  InputSameDT=on
  Sum : Sum  SaturateOnIntegerOverflow=on  InputSameDT=on
  Sum1 : Sum  Inputs=+-  SaturateOnIntegerOverflow=on  InputSameDT=on
  Peo : Outport
  Qeo : Outport  Port=2
  wires:
  Demux1/1 -> Product5/2, Product2/2
  Iq/1 -> Demux1/1
  Gain1/1 -> Qeo/1
  Gain/1 -> Peo/1
  Product2/1 -> Sum/1
  Product3/1 -> Sum/2
  Product4/1 -> Sum1/1
  Product5/1 -> Sum1/2
  Sum/1 -> Gain/1  "Peo"
  Sum1/1 -> Gain1/1  "Qeo"
  Vd/1 -> Product3/1, Product5/1
  Vq/1 -> Product2/1, Product4/1
  Demux1/2 -> Product3/2, Product4/2

== system powerlib_modelsV2/Discrete/synchronous_machine/Subsystem ==
  Vf : Inport  Port=1  LatchInput=off
  Constant : Constant  Value=excAxis
  Ground2 : Ground
  Switch : Switch  Threshold=1.5  InputSameDT=on
  Switch1 : Switch  Threshold=1.5  InputSameDT=on
  Vkq1 : Outport
  Vfd : Outport  Port=2
  wires:
  Switch/1 -> Vkq1/1
  Switch1/1 -> Vfd/1
  Constant/1 -> Switch1/2, Switch/2
  Vf/1 -> Switch/1, Switch1/3
  Ground2/1 -> Switch/3, Switch1/1

== system powerlib_modelsV2/Discrete/synchronous_machine/abc2qd ==
  note: This subsystem converts Vab and Vbc to Vd,Vq. The sine and cosine com-
      | puted here are sent to the inverse transformation subsystem qd/abc.
  v : Inport  Port=1  LatchInput=off
  theta : Inport  Port=2  LatchInput=off
  1_Vb : Gain  Gain=1/Vb  SaturateOnIntegerOverflow=on
  Elementary Math : ElementaryMath
  Elementary Math1 : ElementaryMath  Operator=cos
  Fcn2 : Fcn  Expr=(u[4]*(2*u[1]+u[2]) + (sqrt3*u[2]*u[3])) * one_third
  Fcn3 : Fcn  Expr=(u[3]*(2*u[1]+u[2]) + (-sqrt3*u[2]*u[4])) * one_third
  Mux1 : Mux  Inputs=[ 2 2 ]
  Mux2 : Mux  Orientation=down  Inputs=[ 1 1 ]
  Mux3 : Mux  Inputs=2
  cos,sin : Outport  InitialOutput=0
  vq : Outport  Port=2  InitialOutput=0
  vd : Outport  Port=3  InitialOutput=0
  vq,vd : Outport  Port=4  InitialOutput=0
  wires:
  Fcn3/1 -> Mux2/2, vd/1
  Fcn2/1 -> Mux2/1, vq/1
  Elementary Math1/1 -> Mux3/2
  Elementary Math/1 -> Mux3/1
  theta/1 -> Elementary Math1/1, Elementary Math/1
  Mux3/1 -> cos,sin/1, Mux1/2
  Mux1/1 -> Fcn3/1, Fcn2/1
  v/1 -> 1_Vb/1
  1_Vb/1 -> Mux1/1
  Mux2/1 -> vq,vd/1

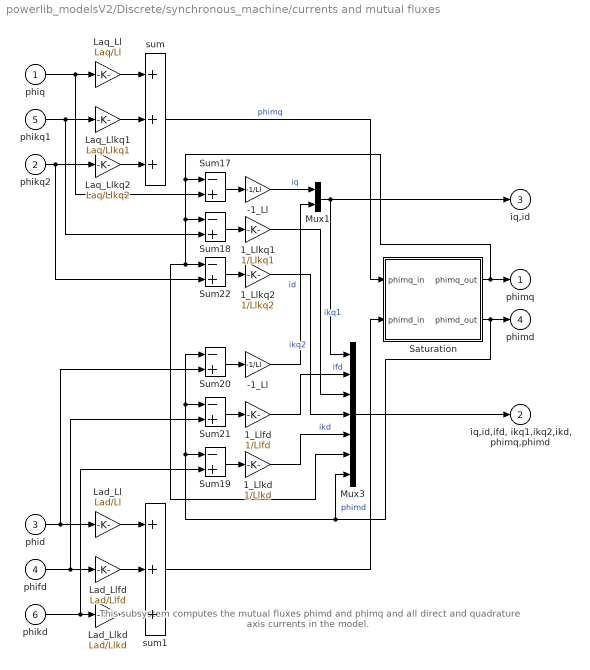
== system powerlib_modelsV2/Discrete/synchronous_machine/currents and mutual fluxes ==
  note: This subsystem computes the mutual fluxes phimd
      | and phimq and all direct and quadrature axis
      | currents in the model.
  phiq : Inport  Port=1  LatchInput=off
  phikq2 : Inport  Port=2  LatchInput=off
  phid : Inport  Port=3  LatchInput=off
  phifd : Inport  Port=4  LatchInput=off
  phikq1 : Inport  Port=5  LatchInput=off
  phikd : Inport  Port=6  LatchInput=off
  -1_Ll : Gain  Gain=-1/Ll  SaturateOnIntegerOverflow=on
  "-1_Ll " : Gain  Gain=-1/Ll  SaturateOnIntegerOverflow=on
  1_Llfd : Gain  Gain=1/Llfd  SaturateOnIntegerOverflow=on
  1_Llkd : Gain  Gain=1/Llkd  SaturateOnIntegerOverflow=on
  1_Llkq1 : Gain  Gain=1/Llkq1  SaturateOnIntegerOverflow=on
  1_Llkq2 : Gain  Gain=1/Llkq2  SaturateOnIntegerOverflow=on
  Lad_Ll : Gain  Gain=Lad/Ll  SaturateOnIntegerOverflow=on
  Lad_Llfd : Gain  Gain=Lad/Llfd  SaturateOnIntegerOverflow=on
  Lad_Llkd : Gain  Gain=Lad/Llkd  SaturateOnIntegerOverflow=on
  Laq_Ll : Gain  Gain=Laq/Ll  SaturateOnIntegerOverflow=on
  Laq_Llkq1 : Gain  Gain=Laq/Llkq1  SaturateOnIntegerOverflow=on
  Laq_Llkq2 : Gain  Gain=Laq/Llkq2  SaturateOnIntegerOverflow=on
  Mux1 : Mux  Inputs=2
  Mux3 : Mux  Inputs=[2 1 1 1 1 1 1]
  Saturation : Subsystem
  Sum{17..22} (6 alike) : Sum  Inputs=-+  SaturateOnIntegerOverflow=on  InputSameDT=on
  sum : Sum  Inputs=+++  SaturateOnIntegerOverflow=on  InputSameDT=on
  sum1 : Sum  Inputs=+++  SaturateOnIntegerOverflow=on  InputSameDT=on
  phimq : Outport  InitialOutput=0
  "iq,id,ifd, ikq1,ikq2,ikd, phimq,phimd" : Outport  Port=2  InitialOutput=0
  iq,id : Outport  Port=3  InitialOutput=0
  phimd : Outport  Port=4  InitialOutput=0
  wires:
  phikq1/1 -> Sum18/2, Laq_Llkq1/1
  phikq2/1 -> Sum22/2, Laq_Llkq2/1
  Laq_Llkq1/1 -> sum/2
  Laq_Llkq2/1 -> sum/3
  Laq_Ll/1 -> sum/1
  phiq/1 -> Sum17/2, Laq_Ll/1
  phikd/1 -> Sum19/2, Lad_Llkd/1
  phid/1 -> Lad_Ll/1, Sum20/2
  phifd/1 -> Sum21/2, Lad_Llfd/1
  Lad_Ll/1 -> sum1/1
  Lad_Llfd/1 -> sum1/2
  Lad_Llkd/1 -> sum1/3
  Mux1/1 -> Mux3/1, iq,id/1
  -1_Ll/1 -> Mux1/1  "iq"
  Sum22/1 -> 1_Llkq2/1
  Sum17/1 -> -1_Ll/1
  Sum18/1 -> 1_Llkq1/1
  1_Llkd/1 -> Mux3/5  "ikd"
  1_Llfd/1 -> Mux3/2  "ifd"
  Sum19/1 -> 1_Llkd/1
  Sum21/1 -> 1_Llfd/1
  "-1_Ll "/1 -> Mux1/2  "id"
  Sum20/1 -> "-1_Ll "/1
  1_Llkq1/1 -> Mux3/3  "ikq1"
  1_Llkq2/1 -> Mux3/4  "ikq2"
  Mux3/1 -> "iq,id,ifd, ikq1,ikq2,ikd, phimq,phimd"/1
  sum/1 -> Saturation/1(phimq_in)  "phimq"
  sum1/1 -> Saturation/2(phimd_in)  "phimd"
  Saturation/1(phimq_out) -> phimq/1, Sum18/1, Sum22/1, Mux3/6, Sum17/1
  Saturation/2(phimd_out) -> phimd/1, Sum20/1, Sum21/1, Sum19/1, Mux3/7

== system powerlib_modelsV2/Discrete/synchronous_machine/mec ==
  note: This subsystem models the mechanical part of the machine.
  "iq,id " : Inport  Port=1  LatchInput=off
  phid : Inport  Port=2  LatchInput=off
  phiq : Inport  Port=3  LatchInput=off
  Pm : Inport  Port=4  LatchInput=off
  1_(2H) : Gain  Gain=1/(2*H)  SaturateOnIntegerOverflow=on
  1_Pb : Gain  Gain=1/Pb  SaturateOnIntegerOverflow=on
  Clock : Clock
      settings: Decimation=10
  Discrete-Time Integrator : DiscreteIntegrator  InitialCondition=dwo  SampleTime=Ts  SaturateOnIntegerOverflow=on  ICPrevOutput=DiscIntNeverNeededParam  ICPrevScaledInput=DiscIntNeverNeededParam
  Discrete-Time Integrator1 : DiscreteIntegrator  InitialCondition=tho  SampleTime=Ts  SaturateOnIntegerOverflow=on  ICPrevOutput=DiscIntNeverNeededParam  ICPrevScaledInput=DiscIntNeverNeededParam
  F : Gain  Orientation=left  Gain=F  SaturateOnIntegerOverflow=on
  Mux : Mux  Inputs=[ 1 1 2 ]
  Mux1 : Mux  Inputs=2
  Mux2 : Mux
  Product : Product  SaturateOnIntegerOverflow=on  InputSameDT=on
  Sum : Sum  SaturateOnIntegerOverflow=on  InputSameDT=on
  Sum2 : Sum  Inputs=+--  SaturateOnIntegerOverflow=on  InputSameDT=on
  Sum3 : Sum  SaturateOnIntegerOverflow=on  InputSameDT=on
  Te : Fcn  Expr=u[1]*u[3]-u[2]*u[4]
  div : Fcn  Expr=u[2]/u[1]
      mask Display: disp('/')
  nom. speed : Constant
  web1 : Gain  Gain=web_psb  SaturateOnIntegerOverflow=on
  web2 : Gain  Gain=web_psb  SaturateOnIntegerOverflow=on
  misc : Outport  InitialOutput=0
  thetae : Outport  Port=2  InitialOutput=0
  we : Outport  Port=3  InitialOutput=0
  "Te " : Outport  Port=4  InitialOutput=0
  wires:
  Sum3/1 -> thetae/1
  Mux2/1 -> misc/1
  Sum/1 -> Mux1/1, we/1, Product/1, Mux2/2  "n"
  Sum2/1 -> 1_(2H)/1
  F/1 -> Sum2/3
  1_Pb/1 -> Mux1/2
  Pm/1 -> 1_Pb/1
  Mux1/1 -> div/1
  Mux/1 -> Te/1
  Te/1 -> Sum2/2, Product/2, "Te "/1
  "iq,id "/1 -> Mux/3
  phid/1 -> Mux/1
  phiq/1 -> Mux/2
  div/1 -> Sum2/1
  1_(2H)/1 -> Discrete-Time Integrator/1
  nom. speed/1 -> Sum/1
  Product/1 -> Mux2/3  "Pe"
  Discrete-Time Integrator/1 -> Sum/2, Mux2/4, F/1, web1/1  "dw"
  web1/1 -> Discrete-Time Integrator1/1
  Clock/1 -> web2/1
  web2/1 -> Sum3/2
  Discrete-Time Integrator1/1 -> Sum3/1, Mux2/1  "d_theta (rad)"

== system powerlib_modelsV2/Discrete/synchronous_machine/phid ==
  note: This subsystem computes the direct axis flux phid.
  w : Inport  Port=1  LatchInput=off
  phiq : Inport  Port=2  LatchInput=off
  vd : Inport  Port=3  LatchInput=off
  phimd : Inport  Port=4  LatchInput=off
  Discrete-Time Integrator : DiscreteIntegrator  IntegratorMethod=Integration: Trapezoidal  InitialCondition=phido  SampleTime=Ts  SaturateOnIntegerOverflow=on  ICPrevOutput=DiscIntNeverNeededParam  ICPrevScaledInput=DiscIntNeverNeededParam
  Product1 : Product  SaturateOnIntegerOverflow=on  InputSameDT=on
  Rs_Ll : Gain  Gain=Rs/Ll  SaturateOnIntegerOverflow=on
  Sum2 : Sum  Inputs=+++  SaturateOnIntegerOverflow=on  InputSameDT=on
  Sum9 : Sum  Inputs=+-  SaturateOnIntegerOverflow=on  InputSameDT=on
  Unit Delay1 : UnitDelay  X0=phido  SampleTime=Ts
  web_psb : Gain  Gain=web_psb  SaturateOnIntegerOverflow=on
  phid : Outport  InitialOutput=0
  wires:
  Discrete-Time Integrator/1 -> Unit Delay1/1
  web_psb/1 -> Discrete-Time Integrator/1
  Sum2/1 -> web_psb/1
  Rs_Ll/1 -> Sum2/3
  Sum9/1 -> Rs_Ll/1
  Product1/1 -> Sum2/1
  w/1 -> Product1/1
  phiq/1 -> Product1/2
  vd/1 -> Sum2/2
  phimd/1 -> Sum9/1
  Unit Delay1/1 -> phid/1, Sum9/2

== system powerlib_modelsV2/Discrete/synchronous_machine/phifd ==
  note: This subsystem computes the field flux phifd.
  vfd : Inport  Port=1  LatchInput=off
  phimd : Inport  Port=2  LatchInput=off
  Discrete-Time Integrator : DiscreteIntegrator  IntegratorMethod=Integration: Trapezoidal  InitialCondition=phifdo  SampleTime=Ts  SaturateOnIntegerOverflow=on  ICPrevOutput=DiscIntNeverNeededParam  ICPrevScaledInput=DiscIntNeverNeededParam
  N : Gain  Gain=N  SaturateOnIntegerOverflow=on
  Rf_Llfd : Gain  Gain=Rf/Llfd  SaturateOnIntegerOverflow=on
  Sum10 : Sum  Inputs=+-  SaturateOnIntegerOverflow=on  InputSameDT=on
  Sum3 : Sum  SaturateOnIntegerOverflow=on  InputSameDT=on
  Unit Delay : UnitDelay  Orientation=left  X0=phifdo  SampleTime=Ts
  web_psb : Gain  Gain=web_psb  SaturateOnIntegerOverflow=on
  phifd : Outport  InitialOutput=0
  wires:
  Sum3/1 -> web_psb/1
  Discrete-Time Integrator/1 -> phifd/1, Unit Delay/1
  web_psb/1 -> Discrete-Time Integrator/1
  phimd/1 -> Sum10/1
  Sum10/1 -> Rf_Llfd/1
  Rf_Llfd/1 -> Sum3/2
  vfd/1 -> N/1
  N/1 -> Sum3/1
  Unit Delay/1 -> Sum10/2

== system powerlib_modelsV2/Discrete/synchronous_machine/phikd ==
  note: This subsystem computes the direct axis damper flux phikd.
  phimd : Inport  Port=1  LatchInput=off
  vkd : Inport  Port=2  LatchInput=off
  Discrete-Time Integrator : DiscreteIntegrator  IntegratorMethod=Integration: Trapezoidal  InitialCondition=phikdo  SampleTime=Ts  SaturateOnIntegerOverflow=on  ICPrevOutput=DiscIntNeverNeededParam  ICPrevScaledInput=DiscIntNeverNeededParam
  Rkd_Llkd : Gain  Gain=Rkd/Llkd  SaturateOnIntegerOverflow=on
  Sum11 : Sum  Inputs=-+  SaturateOnIntegerOverflow=on  InputSameDT=on
  Sum4 : Sum  SaturateOnIntegerOverflow=on  InputSameDT=on
  Unit Delay : UnitDelay  Orientation=left  X0=phikdo  SampleTime=Ts
  web_psb : Gain  Gain=web_psb  SaturateOnIntegerOverflow=on
  phikd : Outport  InitialOutput=0
  wires:
  Sum4/1 -> web_psb/1
  Discrete-Time Integrator/1 -> phikd/1, Unit Delay/1
  web_psb/1 -> Discrete-Time Integrator/1
  vkd/1 -> Sum4/2
  phimd/1 -> Sum11/2
  Sum11/1 -> Rkd_Llkd/1
  Rkd_Llkd/1 -> Sum4/1
  Unit Delay/1 -> Sum11/1

== system powerlib_modelsV2/Discrete/synchronous_machine/phikq1 ==
  note: This subsystem computes the quadrature axis damper flux phikq.
  phimq : Inport  Port=1  LatchInput=off
  vkq1 : Inport  Port=2  LatchInput=off
  Discrete-Time Integrator : DiscreteIntegrator  IntegratorMethod=Integration: Trapezoidal  InitialCondition=phikq1o  SampleTime=Ts  SaturateOnIntegerOverflow=on  ICPrevOutput=DiscIntNeverNeededParam  ICPrevScaledInput=DiscIntNeverNeededParam
  Rkq1_Llkq1 : Gain  Gain=Rkq1/Llkq1  SaturateOnIntegerOverflow=on
  Sum1 : Sum  SaturateOnIntegerOverflow=on  InputSameDT=on
  Sum7 : Sum  Inputs=-+  SaturateOnIntegerOverflow=on  InputSameDT=on
  Unit Delay : UnitDelay  Orientation=left  X0=phikq1o  SampleTime=Ts
  web_psb : Gain  Gain=web_psb  SaturateOnIntegerOverflow=on
  phikq1 : Outport  InitialOutput=0
  wires:
  Rkq1_Llkq1/1 -> Sum1/1
  Sum7/1 -> Rkq1_Llkq1/1
  Sum1/1 -> web_psb/1
  phimq/1 -> Sum7/2
  vkq1/1 -> Sum1/2
  web_psb/1 -> Discrete-Time Integrator/1
  Discrete-Time Integrator/1 -> phikq1/1, Unit Delay/1
  Unit Delay/1 -> Sum7/1

== system powerlib_modelsV2/Discrete/synchronous_machine/phikq2 ==
  note: This subsystem computes the quadrature axis damper flux phikq2.
  vkq2 : Inport  Port=1  LatchInput=off
  phimq : Inport  Port=2  LatchInput=off
  Enabled integrator : Subsystem  TreatAsAtomicUnit=on
      mask Display: disp('1/s')
  Rkq2_Llkq2 : Gain  Gain=Rkq2/Llkq2  SaturateOnIntegerOverflow=on
  Sum1 : Sum  SaturateOnIntegerOverflow=on  InputSameDT=on
  Sum7 : Sum  Inputs=-+  SaturateOnIntegerOverflow=on  InputSameDT=on
  Unit Delay : UnitDelay  Orientation=left  X0=phikq2o  SampleTime=Ts
  web_psb : Gain  Gain=web_psb  SaturateOnIntegerOverflow=on
  wref : Constant  Value=isfinite(Llkq2)
  phikq2 : Outport  InitialOutput=0
  wires:
  phimq/1 -> Sum7/2
  Sum1/1 -> web_psb/1
  Rkq2_Llkq2/1 -> Sum1/1
  vkq2/1 -> Sum1/2
  Sum7/1 -> Rkq2_Llkq2/1
  web_psb/1 -> Enabled integrator/1(In1)
  Enabled integrator/1(Out1) -> phikq2/1, Unit Delay/1
  wref/1 -> Enabled integrator/Enable
  Unit Delay/1 -> Sum7/1
